simulink model "KALMANCE"  (R2019b)
settings: Solver=VariableStepAuto  StartTime=0.0  StopTime=10.0  RelTol=1e-3
values from neighbouring files (symbols this model uses):
  Ace = [(A-B*K) (B*K) ... (first row only)    [State_Space.m]
  Bce = [B*Nbar ... (first row only)    [State_Space.m]
  Cce = [Cc zeros(size(Cc))]    [State_Space.m]
  Dce = [0;0]    [State_Space.m]
  K = lqr(A,B,Q,R)    [LQG.m]    (also in State_Space.m; frequency_domain.m = 35; root_locus_method.m = 20; rscale.m = k)
  Nbar = rscale(sys_ss,K)    [State_Space.m]    (also in rscale.m = Nu + K*Nx)
undefined symbols (not defined in the file or in its folder): Ke
settings Model: Creator=Khojasteh Mirza  LastModifiedBy=Khojasteh Mirza

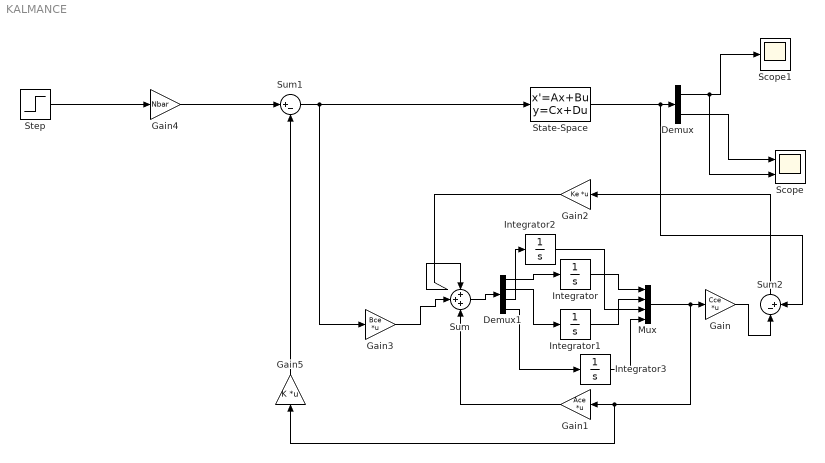
== system KALMANCE ==
  Demux : Demux  Outputs=2
  Demux1 : Demux
  Gain : Gain  Gain=Cce  Multiplication=Matrix(K*u)
  Gain1 : Gain  Gain=Ace  Multiplication=Matrix(K*u)
  Gain2 : Gain  Gain=Ke  Multiplication=Matrix(K*u)
  Gain3 : Gain  Gain=Bce  Multiplication=Matrix(K*u)
  Gain4 : Gain  Gain=Nbar
  Gain5 : Gain  Gain=K  Multiplication=Matrix(K*u)
  Integrator{,1..3} (4 alike) : Integrator
  Mux : Mux
  Scope : Scope  NumInputPorts=2
  Scope1 : Scope
  State-Space : StateSpace  A=Ace  B=Bce  C=Cce  D=Dce  InitialCondition=0
  Step : Step  After=0.5  SampleTime=0
  Sum : Sum  Inputs=3
  Sum1 : Sum  Inputs=|+-
  Sum2 : Sum  Inputs=|-+
  wires:
  Gain3/1 -> Sum/2
  Gain4/1 -> Sum1/1
  Sum/1 -> Demux1/1
  Demux1/1 -> Integrator/1
  Gain1/1 -> Sum/3
  Gain2/1 -> Sum/1
  Sum1/1 -> Gain3/1, State-Space/1
  Gain5/1 -> Sum1/2
  Integrator1/1 -> Mux/2
  State-Space/1 -> Sum2/2, Demux/1
  Demux/1 -> Scope/2, Scope1/1
  Gain/1 -> Sum2/1
  Step/1 -> Gain4/1
  Sum2/1 -> Gain2/1
  Mux/1 -> Gain5/1, Gain1/1, Gain/1
  Demux/2 -> Scope/1
  Demux1/2 -> Integrator1/1
  Integrator/1 -> Mux/1
  Integrator2/1 -> Mux/3
  Demux1/3 -> Integrator2/1
  Demux1/4 -> Integrator3/1
  Integrator3/1 -> Mux/4
